simulink model "HLSDem_SelectParameter"  (R2016b)
settings: configuration reference "CodeGenConfigSet" (kept outside this file)
values from neighbouring files (symbols this model uses):
  HLSDem_facFdbkLoGrip_C = Calibration.Parameter    [init_HLSDem_SelectParameter.m]    (also in init_HLSDem_SelectParameter_SIL.m = Simulink.Parameter)
  HLSDem_facFdbkLoNoGrip_C = Calibration.Parameter    [init_HLSDem_SelectParameter.m]    (also in init_HLSDem_SelectParameter_SIL.m = Simulink.Parameter)
  HLSDem_facFdbkTrqLosHiGrip_CUR = Calibration.Parameter    [init_HLSDem_SelectParameter.m]    (also in init_HLSDem_SelectParameter_SIL.m = Simulink.Parameter)
  HLSDem_facFdbkTrqLosHiGrip_CURX = Calibration.Parameter    [init_HLSDem_SelectParameter.m]    (also in init_HLSDem_SelectParameter_SIL.m = Simulink.Parameter)
  HLSDem_facFdbkTrqLosHiNoGrip_C = Calibration.Parameter    [init_HLSDem_SelectParameter.m]    (also in init_HLSDem_SelectParameter_SIL.m = Simulink.Parameter)
  HLSDem_facFdbkTrqLosLoGrip_CUR = Calibration.Parameter    [init_HLSDem_SelectParameter.m]    (also in init_HLSDem_SelectParameter_SIL.m = Simulink.Parameter)
  HLSDem_facFdbkTrqLosLoGrip_CURX = Calibration.Parameter    [init_HLSDem_SelectParameter.m]    (also in init_HLSDem_SelectParameter_SIL.m = Simulink.Parameter)
  HLSDem_facFdbkTrqLosLoNoGrip_C = Calibration.Parameter    [init_HLSDem_SelectParameter.m]    (also in init_HLSDem_SelectParameter_SIL.m = Simulink.Parameter)
  HLSDem_facNAvrgPT1_C = Calibration.Parameter    [init_HLSDem_SelectParameter.m]    (also in init_HLSDem_SelectParameter_SIL.m = Simulink.Parameter)
  HLSDem_facTrqPT1CorFac_C = Calibration.Parameter    [init_HLSDem_SelectParameter.m]    (also in init_HLSDem_SelectParameter_SIL.m = Simulink.Parameter)
  HLSDem_GripIKiHi_CUR = Calibration.Parameter    [init_HLSDem_SelectParameter.m]    (also in init_HLSDem_SelectParameter_SIL.m = Simulink.Parameter)
  HLSDem_GripIKiHi_CURX = Calibration.Parameter    [init_HLSDem_SelectParameter.m]    (also in init_HLSDem_SelectParameter_SIL.m = Simulink.Parameter)
  HLSDem_GripIKiLo_CUR = Calibration.Parameter    [init_HLSDem_SelectParameter.m]    (also in init_HLSDem_SelectParameter_SIL.m = Simulink.Parameter)
  HLSDem_GripIKiLo_CURX = Calibration.Parameter    [init_HLSDem_SelectParameter.m]    (also in init_HLSDem_SelectParameter_SIL.m = Simulink.Parameter)
  HLSDem_GripIKiNegHi_CUR = Calibration.Parameter    [init_HLSDem_SelectParameter.m]    (also in init_HLSDem_SelectParameter_SIL.m = Simulink.Parameter)
  HLSDem_GripIKiNegHi_CURX = Calibration.Parameter    [init_HLSDem_SelectParameter.m]    (also in init_HLSDem_SelectParameter_SIL.m = Simulink.Parameter)
  HLSDem_GripIKiNegLo_CUR = Calibration.Parameter    [init_HLSDem_SelectParameter.m]    (also in init_HLSDem_SelectParameter_SIL.m = Simulink.Parameter)
  HLSDem_GripIKiNegLo_CURX = Calibration.Parameter    [init_HLSDem_SelectParameter.m]    (also in init_HLSDem_SelectParameter_SIL.m = Simulink.Parameter)
  HLSDem_GripIKiPosHi_CUR = Calibration.Parameter    [init_HLSDem_SelectParameter.m]    (also in init_HLSDem_SelectParameter_SIL.m = Simulink.Parameter)
  HLSDem_GripIKiPosHi_CURX = Calibration.Parameter    [init_HLSDem_SelectParameter.m]    (also in init_HLSDem_SelectParameter_SIL.m = Simulink.Parameter)
  HLSDem_GripIKiPosLo_CUR = Calibration.Parameter    [init_HLSDem_SelectParameter.m]    (also in init_HLSDem_SelectParameter_SIL.m = Simulink.Parameter)
  HLSDem_GripIKiPosLo_CURX = Calibration.Parameter    [init_HLSDem_SelectParameter.m]    (also in init_HLSDem_SelectParameter_SIL.m = Simulink.Parameter)
  HLSDem_GripIWinNegHi_C = Calibration.Parameter    [init_HLSDem_SelectParameter.m]    (also in init_HLSDem_SelectParameter_SIL.m = Simulink.Parameter)
  HLSDem_GripIWinNegLo_C = Calibration.Parameter    [init_HLSDem_SelectParameter.m]    (also in init_HLSDem_SelectParameter_SIL.m = Simulink.Parameter)
  HLSDem_GripIWinPosHi_C = Calibration.Parameter    [init_HLSDem_SelectParameter.m]    (also in init_HLSDem_SelectParameter_SIL.m = Simulink.Parameter)
  HLSDem_GripIWinPosLo_C = Calibration.Parameter    [init_HLSDem_SelectParameter.m]    (also in init_HLSDem_SelectParameter_SIL.m = Simulink.Parameter)
  HLSDem_GripPKpHi_CUR = Calibration.Parameter    [init_HLSDem_SelectParameter.m]    (also in init_HLSDem_SelectParameter_SIL.m = Simulink.Parameter)
  HLSDem_GripPKpHi_CURX = Calibration.Parameter    [init_HLSDem_SelectParameter.m]    (also in init_HLSDem_SelectParameter_SIL.m = Simulink.Parameter)
  HLSDem_GripPKpLo_CUR = Calibration.Parameter    [init_HLSDem_SelectParameter.m]    (also in init_HLSDem_SelectParameter_SIL.m = Simulink.Parameter)
  HLSDem_GripPKpLo_CURX = Calibration.Parameter    [init_HLSDem_SelectParameter.m]    (also in init_HLSDem_SelectParameter_SIL.m = Simulink.Parameter)
  HLSDem_GripPKpNegHi_CUR = Calibration.Parameter    [init_HLSDem_SelectParameter.m]    (also in init_HLSDem_SelectParameter_SIL.m = Simulink.Parameter)
  HLSDem_GripPKpNegHi_CURX = Calibration.Parameter    [init_HLSDem_SelectParameter.m]    (also in init_HLSDem_SelectParameter_SIL.m = Simulink.Parameter)
  HLSDem_GripPKpNegLo_CUR = Calibration.Parameter    [init_HLSDem_SelectParameter.m]    (also in init_HLSDem_SelectParameter_SIL.m = Simulink.Parameter)
  HLSDem_GripPKpNegLo_CURX = Calibration.Parameter    [init_HLSDem_SelectParameter.m]    (also in init_HLSDem_SelectParameter_SIL.m = Simulink.Parameter)
  HLSDem_GripPKpPosHi_CUR = Calibration.Parameter    [init_HLSDem_SelectParameter.m]    (also in init_HLSDem_SelectParameter_SIL.m = Simulink.Parameter)
  HLSDem_GripPKpPosHi_CURX = Calibration.Parameter    [init_HLSDem_SelectParameter.m]    (also in init_HLSDem_SelectParameter_SIL.m = Simulink.Parameter)
  HLSDem_GripPKpPosLo_CUR = Calibration.Parameter    [init_HLSDem_SelectParameter.m]    (also in init_HLSDem_SelectParameter_SIL.m = Simulink.Parameter)
  HLSDem_GripPKpPosLo_CURX = Calibration.Parameter    [init_HLSDem_SelectParameter.m]    (also in init_HLSDem_SelectParameter_SIL.m = Simulink.Parameter)
  HLSDem_GripPWinNegHi_C = Calibration.Parameter    [init_HLSDem_SelectParameter.m]    (also in init_HLSDem_SelectParameter_SIL.m = Simulink.Parameter)
  HLSDem_GripPWinNegLo_C = Calibration.Parameter    [init_HLSDem_SelectParameter.m]    (also in init_HLSDem_SelectParameter_SIL.m = Simulink.Parameter)
  HLSDem_GripPWinPosHi_C = Calibration.Parameter    [init_HLSDem_SelectParameter.m]    (also in init_HLSDem_SelectParameter_SIL.m = Simulink.Parameter)
  HLSDem_GripPWinPosLo_C = Calibration.Parameter    [init_HLSDem_SelectParameter.m]    (also in init_HLSDem_SelectParameter_SIL.m = Simulink.Parameter)
  HLSDem_InrtVehGrip_CUR = Calibration.Parameter    [init_HLSDem_SelectParameter.m]    (also in init_HLSDem_SelectParameter_SIL.m = Simulink.Parameter)
  HLSDem_InrtVehGrip_CURX = Calibration.Parameter    [init_HLSDem_SelectParameter.m]    (also in init_HLSDem_SelectParameter_SIL.m = Simulink.Parameter)
  HLSDem_InrtVehNoGrip_C = Calibration.Parameter    [init_HLSDem_SelectParameter.m]    (also in init_HLSDem_SelectParameter_SIL.m = Simulink.Parameter)
  HLSDem_KiCorFac_MAP = Calibration.Parameter    [init_HLSDem_SelectParameter.m]    (also in init_HLSDem_SelectParameter_SIL.m = Simulink.Parameter)
  HLSDem_KiCorFac_MAPX = Calibration.Parameter    [init_HLSDem_SelectParameter.m]    (also in init_HLSDem_SelectParameter_SIL.m = Simulink.Parameter)
  HLSDem_KiCorFac_MAPY = Calibration.Parameter    [init_HLSDem_SelectParameter.m]    (also in init_HLSDem_SelectParameter_SIL.m = Simulink.Parameter)
  HLSDem_KiCorTrqFac_MAP = Calibration.Parameter    [init_HLSDem_SelectParameter.m]    (also in init_HLSDem_SelectParameter_SIL.m = Simulink.Parameter)
  HLSDem_KiCorTrqFac_MAPX = Calibration.Parameter    [init_HLSDem_SelectParameter.m]    (also in init_HLSDem_SelectParameter_SIL.m = Simulink.Parameter)
  HLSDem_KiCorTrqFac_MAPY = Calibration.Parameter    [init_HLSDem_SelectParameter.m]    (also in init_HLSDem_SelectParameter_SIL.m = Simulink.Parameter)
  HLSDem_KpCorFac_MAP = Calibration.Parameter    [init_HLSDem_SelectParameter.m]    (also in init_HLSDem_SelectParameter_SIL.m = Simulink.Parameter)
  HLSDem_KpCorFac_MAPX = Calibration.Parameter    [init_HLSDem_SelectParameter.m]    (also in init_HLSDem_SelectParameter_SIL.m = Simulink.Parameter)
  HLSDem_KpCorFac_MAPY = Calibration.Parameter    [init_HLSDem_SelectParameter.m]    (also in init_HLSDem_SelectParameter_SIL.m = Simulink.Parameter)
  HLSDem_KpCorTrqFac_MAP = Calibration.Parameter    [init_HLSDem_SelectParameter.m]    (also in init_HLSDem_SelectParameter_SIL.m = Simulink.Parameter)
  HLSDem_KpCorTrqFac_MAPX = Calibration.Parameter    [init_HLSDem_SelectParameter.m]    (also in init_HLSDem_SelectParameter_SIL.m = Simulink.Parameter)
  HLSDem_KpCorTrqFac_MAPY = Calibration.Parameter    [init_HLSDem_SelectParameter.m]    (also in init_HLSDem_SelectParameter_SIL.m = Simulink.Parameter)
  HLSDem_NoGripdnAccLim_C = Calibration.Parameter    [init_HLSDem_SelectParameter.m]    (also in init_HLSDem_SelectParameter_SIL.m = Simulink.Parameter)
  HLSDem_NoGripdnDeclLim_C = Calibration.Parameter    [init_HLSDem_SelectParameter.m]    (also in init_HLSDem_SelectParameter_SIL.m = Simulink.Parameter)
  HLSDem_NoGripdnDeclLimBrk_C = Calibration.Parameter    [init_HLSDem_SelectParameter.m]    (also in init_HLSDem_SelectParameter_SIL.m = Simulink.Parameter)
  HLSDem_NoGripIKiHi_C = Calibration.Parameter    [init_HLSDem_SelectParameter.m]    (also in init_HLSDem_SelectParameter_SIL.m = Simulink.Parameter)
  HLSDem_NoGripIKiLo_C = Calibration.Parameter    [init_HLSDem_SelectParameter.m]    (also in init_HLSDem_SelectParameter_SIL.m = Simulink.Parameter)
  HLSDem_NoGripIKiNegHi_C = Calibration.Parameter    [init_HLSDem_SelectParameter.m]    (also in init_HLSDem_SelectParameter_SIL.m = Simulink.Parameter)
  HLSDem_NoGripIKiNegLo_C = Calibration.Parameter    [init_HLSDem_SelectParameter.m]    (also in init_HLSDem_SelectParameter_SIL.m = Simulink.Parameter)
  HLSDem_NoGripIKiPosHi_C = Calibration.Parameter    [init_HLSDem_SelectParameter.m]    (also in init_HLSDem_SelectParameter_SIL.m = Simulink.Parameter)
  HLSDem_NoGripIKiPosLo_C = Calibration.Parameter    [init_HLSDem_SelectParameter.m]    (also in init_HLSDem_SelectParameter_SIL.m = Simulink.Parameter)
  HLSDem_NoGripIWinNegHi_C = Calibration.Parameter    [init_HLSDem_SelectParameter.m]    (also in init_HLSDem_SelectParameter_SIL.m = Simulink.Parameter)
  HLSDem_NoGripIWinNegLo_C = Calibration.Parameter    [init_HLSDem_SelectParameter.m]    (also in init_HLSDem_SelectParameter_SIL.m = Simulink.Parameter)
  HLSDem_NoGripIWinPosHi_C = Calibration.Parameter    [init_HLSDem_SelectParameter.m]    (also in init_HLSDem_SelectParameter_SIL.m = Simulink.Parameter)
  HLSDem_NoGripIWinPosLo_C = Calibration.Parameter    [init_HLSDem_SelectParameter.m]    (also in init_HLSDem_SelectParameter_SIL.m = Simulink.Parameter)
  HLSDem_NoGripPKpHi_C = Calibration.Parameter    [init_HLSDem_SelectParameter.m]    (also in init_HLSDem_SelectParameter_SIL.m = Simulink.Parameter)
  HLSDem_NoGripPKpLo_C = Calibration.Parameter    [init_HLSDem_SelectParameter.m]    (also in init_HLSDem_SelectParameter_SIL.m = Simulink.Parameter)
  HLSDem_NoGripPKpNegHi_C = Calibration.Parameter    [init_HLSDem_SelectParameter.m]    (also in init_HLSDem_SelectParameter_SIL.m = Simulink.Parameter)
  HLSDem_NoGripPKpNegLo_C = Calibration.Parameter    [init_HLSDem_SelectParameter.m]    (also in init_HLSDem_SelectParameter_SIL.m = Simulink.Parameter)
  HLSDem_NoGripPKpPosHi_C = Calibration.Parameter    [init_HLSDem_SelectParameter.m]    (also in init_HLSDem_SelectParameter_SIL.m = Simulink.Parameter)
  HLSDem_NoGripPKpPosLo_C = Calibration.Parameter    [init_HLSDem_SelectParameter.m]    (also in init_HLSDem_SelectParameter_SIL.m = Simulink.Parameter)
  HLSDem_NoGripPWinNegHi_C = Calibration.Parameter    [init_HLSDem_SelectParameter.m]    (also in init_HLSDem_SelectParameter_SIL.m = Simulink.Parameter)
  HLSDem_NoGripPWinNegLo_C = Calibration.Parameter    [init_HLSDem_SelectParameter.m]    (also in init_HLSDem_SelectParameter_SIL.m = Simulink.Parameter)
  HLSDem_NoGripPWinPosHi_C = Calibration.Parameter    [init_HLSDem_SelectParameter.m]    (also in init_HLSDem_SelectParameter_SIL.m = Simulink.Parameter)
  HLSDem_NoGripPWinPosLo_C = Calibration.Parameter    [init_HLSDem_SelectParameter.m]    (also in init_HLSDem_SelectParameter_SIL.m = Simulink.Parameter)
  HLSDem_rNoGripThres_C = Calibration.Parameter    [init_HLSDem_SelectParameter.m]    (also in init_HLSDem_SelectParameter_SIL.m = Simulink.Parameter)
  HLSDem_stBrkTrq_C = Calibration.Parameter    [init_HLSDem_SelectParameter.m]    (also in init_HLSDem_SelectParameter_SIL.m = Simulink.Parameter)
  HLSDem_swtTempSelParAdap_C = Calibration.Parameter    [init_HLSDem_SelectParameter.m]    (also in init_HLSDem_SelectParameter_SIL.m = Simulink.Parameter)
  HLSDem_swtTrqSelCorFac_C = Calibration.Parameter    [init_HLSDem_SelectParameter.m]    (also in init_HLSDem_SelectParameter_SIL.m = Simulink.Parameter)
  HLSDem_tiFltTrqLosGrip_CUR = Calibration.Parameter    [init_HLSDem_SelectParameter.m]    (also in init_HLSDem_SelectParameter_SIL.m = Simulink.Parameter)
  HLSDem_tiFltTrqLosGrip_CURX = Calibration.Parameter    [init_HLSDem_SelectParameter.m]    (also in init_HLSDem_SelectParameter_SIL.m = Simulink.Parameter)
  HLSDem_tiFltTrqLosNoGrip_C = Calibration.Parameter    [init_HLSDem_SelectParameter.m]    (also in init_HLSDem_SelectParameter_SIL.m = Simulink.Parameter)
libraries: CXLib x2
(part 2 of 2)

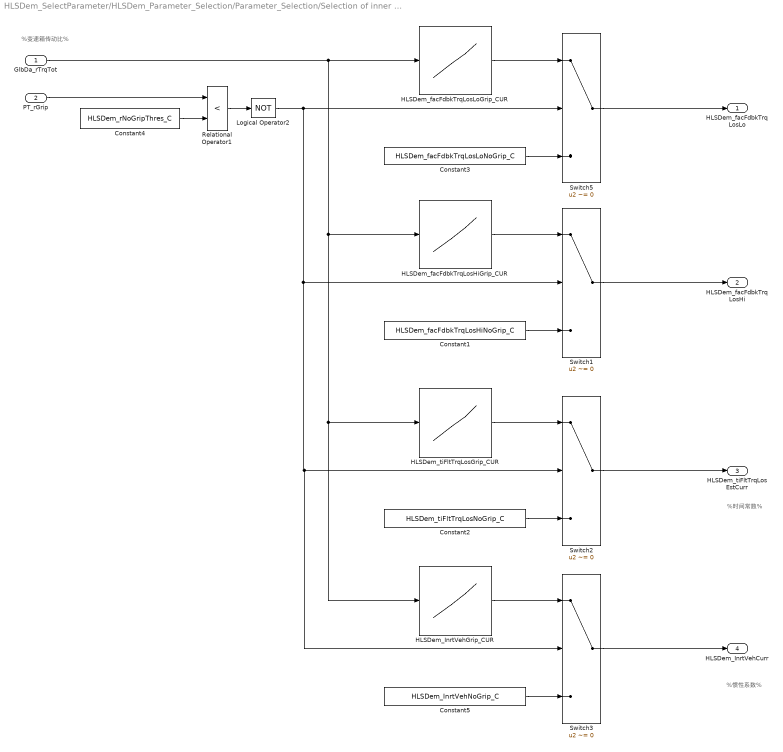
== system HLSDem_SelectParameter/HLSDem_Parameter_Selection/Parameter_Selection/Selection of inner feedback factor ==
  note: %时间常数%
  note: %变速箱传动比%
  note: %惯性系数%
  GlbDa_rTrqTot : Inport
  PT_rGrip : Inport  Port=2
  Constant1 : Constant  Value=HLSDem_facFdbkTrqLosHiNoGrip_C
  Constant2 : Constant  Value=HLSDem_tiFltTrqLosNoGrip_C
  Constant3 : Constant  Value=HLSDem_facFdbkTrqLosLoNoGrip_C
  Constant4 : Constant  Value=HLSDem_rNoGripThres_C
  Constant5 : Constant  Value=HLSDem_InrtVehNoGrip_C
  HLSDem_InrtVehGrip_CUR : Lookup_n-D  NumberOfTableDimensions=1  BreakpointsForDimension1=HLSDem_InrtVehGrip_CURX  BreakpointsForDimension2=HLSDem_KpCorFac_MAPX  Table=HLSDem_InrtVehGrip_CUR  ExtrapMethod=Clip  InternalRulePriority=Speed  OutDataTypeStr=Inherit: Inherit via back propagation  RndMeth=Simplest  SaturateOnIntegerOverflow=on
  HLSDem_facFdbkTrqLosHiGrip_CUR : Lookup_n-D  NumberOfTableDimensions=1  BreakpointsForDimension1=HLSDem_facFdbkTrqLosHiGrip_CURX  BreakpointsForDimension2=HLSDem_KpCorFac_MAPX  Table=HLSDem_facFdbkTrqLosHiGrip_CUR  ExtrapMethod=Clip  InternalRulePriority=Speed  OutDataTypeStr=Inherit: Inherit via back propagation  RndMeth=Simplest  SaturateOnIntegerOverflow=on
  HLSDem_facFdbkTrqLosLoGrip_CUR : Lookup_n-D  NumberOfTableDimensions=1  BreakpointsForDimension1=HLSDem_facFdbkTrqLosLoGrip_CURX  BreakpointsForDimension2=HLSDem_KpCorFac_MAPX  Table=HLSDem_facFdbkTrqLosLoGrip_CUR  ExtrapMethod=Clip  InternalRulePriority=Speed  OutDataTypeStr=Inherit: Inherit via back propagation  RndMeth=Simplest  SaturateOnIntegerOverflow=on
  HLSDem_tiFltTrqLosGrip_CUR : Lookup_n-D  NumberOfTableDimensions=1  BreakpointsForDimension1=HLSDem_tiFltTrqLosGrip_CURX  BreakpointsForDimension2=HLSDem_KpCorFac_MAPX  Table=HLSDem_tiFltTrqLosGrip_CUR  ExtrapMethod=Clip  InternalRulePriority=Speed  OutDataTypeStr=Inherit: Inherit via back propagation  RndMeth=Simplest  SaturateOnIntegerOverflow=on
  Logical Operator2 : Logic  Operator=NOT  AllPortsSameDT=off  OutDataTypeStr=boolean
  Relational Operator1 : RelationalOperator  Operator=<  OutDataTypeStr=boolean  RndMeth=Nearest  InputSameDT=on
  Switch{1..3,5} (4 alike) : Switch  Criteria=u2 ~= 0  InputSameDT=on
  HLSDem_facFdbkTrqLosLo : Outport
  HLSDem_facFdbkTrqLosHi : Outport  Port=2
  HLSDem_tiFltTrqLosEstCurr : Outport  Port=3
  HLSDem_InrtVehCurr : Outport  Port=4
  wires:
  Relational Operator1/1 -> Logical Operator2/1
  Switch2/1 -> HLSDem_tiFltTrqLosEstCurr/1
  GlbDa_rTrqTot/1 -> HLSDem_tiFltTrqLosGrip_CUR/1, HLSDem_InrtVehGrip_CUR/1, HLSDem_facFdbkTrqLosHiGrip_CUR/1, HLSDem_facFdbkTrqLosLoGrip_CUR/1
  Switch1/1 -> HLSDem_facFdbkTrqLosHi/1
  HLSDem_facFdbkTrqLosLoGrip_CUR/1 -> Switch5/1
  PT_rGrip/1 -> Relational Operator1/1
  HLSDem_facFdbkTrqLosHiGrip_CUR/1 -> Switch1/1
  Logical Operator2/1 -> Switch1/2, Switch3/2, Switch2/2, Switch5/2
  Constant3/1 -> Switch5/3
  Constant2/1 -> Switch2/3
  Constant1/1 -> Switch1/3
  Constant5/1 -> Switch3/3
  Switch5/1 -> HLSDem_facFdbkTrqLosLo/1
  HLSDem_tiFltTrqLosGrip_CUR/1 -> Switch2/1
  Constant4/1 -> Relational Operator1/2
  Switch3/1 -> HLSDem_InrtVehCurr/1
  HLSDem_InrtVehGrip_CUR/1 -> Switch3/1

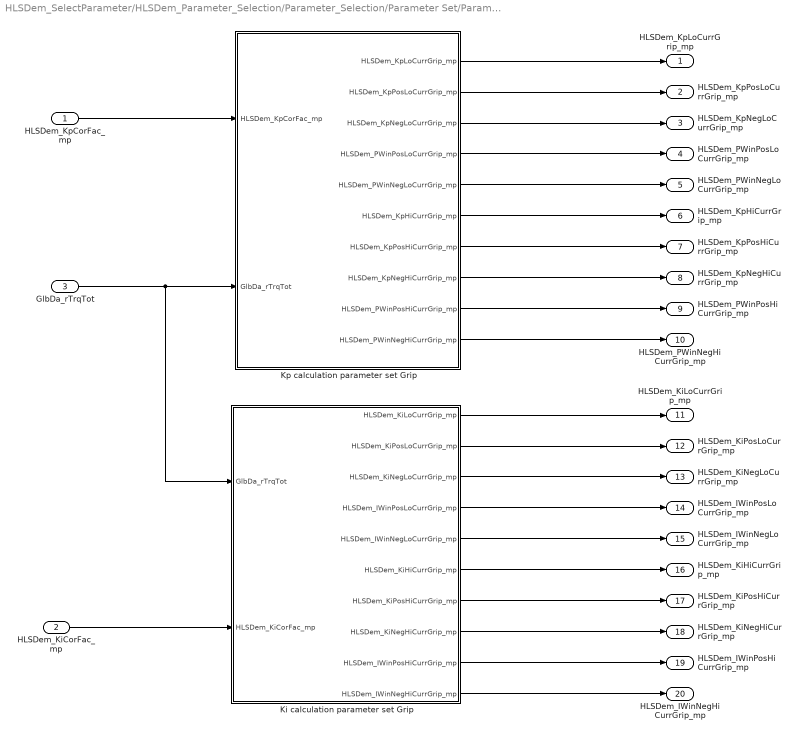
== system HLSDem_SelectParameter/HLSDem_Parameter_Selection/Parameter_Selection/Parameter Set/Parameter set Grip ==
  HLSDem_KpCorFac_mp : Inport
  HLSDem_KiCorFac_mp : Inport  Port=2
  GlbDa_rTrqTot : Inport  Port=3
  Ki calculation parameter set Grip : Subsystem
  Kp calculation parameter set Grip : Subsystem
  HLSDem_KpLoCurrGrip_mp : Outport
  HLSDem_KpPosLoCurrGrip_mp : Outport  Port=2
  HLSDem_KpNegLoCurrGrip_mp : Outport  Port=3
  HLSDem_PWinPosLoCurrGrip_mp : Outport  Port=4
  HLSDem_PWinNegLoCurrGrip_mp : Outport  Port=5
  HLSDem_KpHiCurrGrip_mp : Outport  Port=6
  HLSDem_KpPosHiCurrGrip_mp : Outport  Port=7
  HLSDem_KpNegHiCurrGrip_mp : Outport  Port=8
  HLSDem_PWinPosHiCurrGrip_mp : Outport  Port=9
  HLSDem_PWinNegHiCurrGrip_mp : Outport  Port=10
  HLSDem_KiLoCurrGrip_mp : Outport  Port=11
  HLSDem_KiPosLoCurrGrip_mp : Outport  Port=12
  HLSDem_KiNegLoCurrGrip_mp : Outport  Port=13
  HLSDem_IWinPosLoCurrGrip_mp : Outport  Port=14
  HLSDem_IWinNegLoCurrGrip_mp : Outport  Port=15
  HLSDem_KiHiCurrGrip_mp : Outport  Port=16
  HLSDem_KiPosHiCurrGrip_mp : Outport  Port=17
  HLSDem_KiNegHiCurrGrip_mp : Outport  Port=18
  HLSDem_IWinPosHiCurrGrip_mp : Outport  Port=19
  HLSDem_IWinNegHiCurrGrip_mp : Outport  Port=20
  wires:
  HLSDem_KiCorFac_mp/1 -> Ki calculation parameter set Grip/2(HLSDem_KiCorFac_mp)
  Ki calculation parameter set Grip/3(HLSDem_KiNegLoCurrGrip_mp) -> HLSDem_KiNegLoCurrGrip_mp/1
  Ki calculation parameter set Grip/5(HLSDem_IWinNegLoCurrGrip_mp) -> HLSDem_IWinNegLoCurrGrip_mp/1
  Ki calculation parameter set Grip/2(HLSDem_KiPosLoCurrGrip_mp) -> HLSDem_KiPosLoCurrGrip_mp/1
  Ki calculation parameter set Grip/4(HLSDem_IWinPosLoCurrGrip_mp) -> HLSDem_IWinPosLoCurrGrip_mp/1
  Kp calculation parameter set Grip/2(HLSDem_KpPosLoCurrGrip_mp) -> HLSDem_KpPosLoCurrGrip_mp/1
  Kp calculation parameter set Grip/7(HLSDem_KpPosHiCurrGrip_mp) -> HLSDem_KpPosHiCurrGrip_mp/1
  Kp calculation parameter set Grip/3(HLSDem_KpNegLoCurrGrip_mp) -> HLSDem_KpNegLoCurrGrip_mp/1
  Kp calculation parameter set Grip/6(HLSDem_KpHiCurrGrip_mp) -> HLSDem_KpHiCurrGrip_mp/1
  HLSDem_KpCorFac_mp/1 -> Kp calculation parameter set Grip/1(HLSDem_KpCorFac_mp)
  Kp calculation parameter set Grip/8(HLSDem_KpNegHiCurrGrip_mp) -> HLSDem_KpNegHiCurrGrip_mp/1
  Kp calculation parameter set Grip/5(HLSDem_PWinNegLoCurrGrip_mp) -> HLSDem_PWinNegLoCurrGrip_mp/1
  Kp calculation parameter set Grip/9(HLSDem_PWinPosHiCurrGrip_mp) -> HLSDem_PWinPosHiCurrGrip_mp/1
  Ki calculation parameter set Grip/9(HLSDem_IWinPosHiCurrGrip_mp) -> HLSDem_IWinPosHiCurrGrip_mp/1
  Ki calculation parameter set Grip/6(HLSDem_KiHiCurrGrip_mp) -> HLSDem_KiHiCurrGrip_mp/1
  Kp calculation parameter set Grip/4(HLSDem_PWinPosLoCurrGrip_mp) -> HLSDem_PWinPosLoCurrGrip_mp/1
  GlbDa_rTrqTot/1 -> Ki calculation parameter set Grip/1(GlbDa_rTrqTot), Kp calculation parameter set Grip/2(GlbDa_rTrqTot)
  Kp calculation parameter set Grip/1(HLSDem_KpLoCurrGrip_mp) -> HLSDem_KpLoCurrGrip_mp/1
  Ki calculation parameter set Grip/8(HLSDem_KiNegHiCurrGrip_mp) -> HLSDem_KiNegHiCurrGrip_mp/1
  Ki calculation parameter set Grip/10(HLSDem_IWinNegHiCurrGrip_mp) -> HLSDem_IWinNegHiCurrGrip_mp/1
  Ki calculation parameter set Grip/1(HLSDem_KiLoCurrGrip_mp) -> HLSDem_KiLoCurrGrip_mp/1
  Kp calculation parameter set Grip/10(HLSDem_PWinNegHiCurrGrip_mp) -> HLSDem_PWinNegHiCurrGrip_mp/1
  Ki calculation parameter set Grip/7(HLSDem_KiPosHiCurrGrip_mp) -> HLSDem_KiPosHiCurrGrip_mp/1

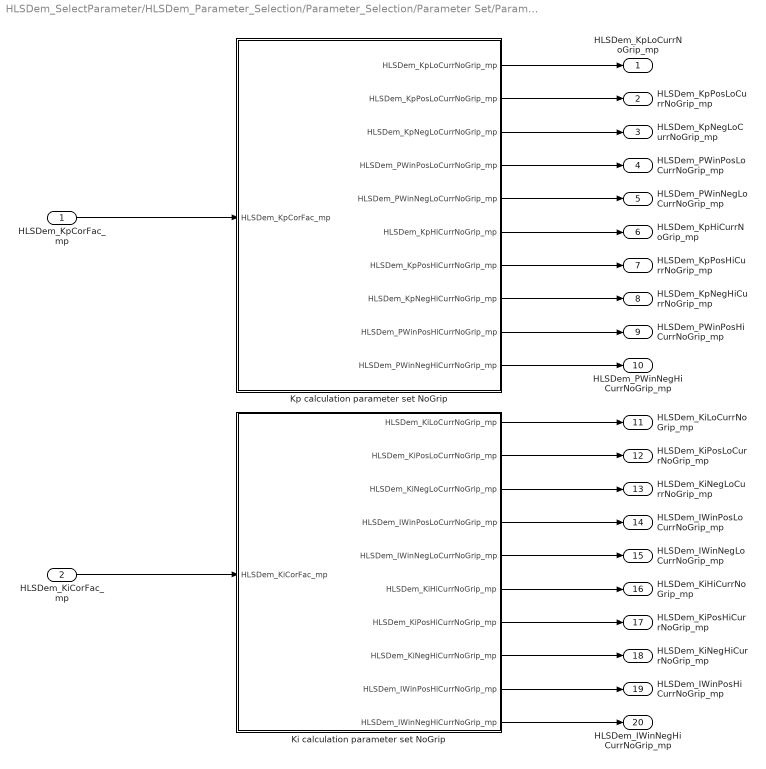
== system HLSDem_SelectParameter/HLSDem_Parameter_Selection/Parameter_Selection/Parameter Set/Parameter set NoGrip  ==
  HLSDem_KpCorFac_mp : Inport
  HLSDem_KiCorFac_mp : Inport  Port=2
  Ki calculation parameter set NoGrip : Subsystem
  Kp calculation parameter set NoGrip : Subsystem
  HLSDem_KpLoCurrNoGrip_mp : Outport
  HLSDem_KpPosLoCurrNoGrip_mp : Outport  Port=2
  HLSDem_KpNegLoCurrNoGrip_mp : Outport  Port=3
  HLSDem_PWinPosLoCurrNoGrip_mp : Outport  Port=4
  HLSDem_PWinNegLoCurrNoGrip_mp : Outport  Port=5
  HLSDem_KpHiCurrNoGrip_mp : Outport  Port=6
  HLSDem_KpPosHiCurrNoGrip_mp : Outport  Port=7
  HLSDem_KpNegHiCurrNoGrip_mp : Outport  Port=8
  HLSDem_PWinPosHiCurrNoGrip_mp : Outport  Port=9
  HLSDem_PWinNegHiCurrNoGrip_mp : Outport  Port=10
  HLSDem_KiLoCurrNoGrip_mp : Outport  Port=11
  HLSDem_KiPosLoCurrNoGrip_mp : Outport  Port=12
  HLSDem_KiNegLoCurrNoGrip_mp : Outport  Port=13
  HLSDem_IWinPosLoCurrNoGrip_mp : Outport  Port=14
  HLSDem_IWinNegLoCurrNoGrip_mp : Outport  Port=15
  HLSDem_KiHiCurrNoGrip_mp : Outport  Port=16
  HLSDem_KiPosHiCurrNoGrip_mp : Outport  Port=17
  HLSDem_KiNegHiCurrNoGrip_mp : Outport  Port=18
  HLSDem_IWinPosHiCurrNoGrip_mp : Outport  Port=19
  HLSDem_IWinNegHiCurrNoGrip_mp : Outport  Port=20
  wires:
  Kp calculation parameter set NoGrip/6(HLSDem_KpHiCurrNoGrip_mp) -> HLSDem_KpHiCurrNoGrip_mp/1
  Kp calculation parameter set NoGrip/7(HLSDem_KpPosHiCurrNoGrip_mp) -> HLSDem_KpPosHiCurrNoGrip_mp/1
  HLSDem_KpCorFac_mp/1 -> Kp calculation parameter set NoGrip/1(HLSDem_KpCorFac_mp)
  Kp calculation parameter set NoGrip/5(HLSDem_PWinNegLoCurrNoGrip_mp) -> HLSDem_PWinNegLoCurrNoGrip_mp/1
  Kp calculation parameter set NoGrip/9(HLSDem_PWinPosHiCurrNoGrip_mp) -> HLSDem_PWinPosHiCurrNoGrip_mp/1
  Kp calculation parameter set NoGrip/1(HLSDem_KpLoCurrNoGrip_mp) -> HLSDem_KpLoCurrNoGrip_mp/1
  Kp calculation parameter set NoGrip/3(HLSDem_KpNegLoCurrNoGrip_mp) -> HLSDem_KpNegLoCurrNoGrip_mp/1
  Kp calculation parameter set NoGrip/8(HLSDem_KpNegHiCurrNoGrip_mp) -> HLSDem_KpNegHiCurrNoGrip_mp/1
  HLSDem_KiCorFac_mp/1 -> Ki calculation parameter set NoGrip/1(HLSDem_KiCorFac_mp)
  Ki calculation parameter set NoGrip/10(HLSDem_IWinNegHiCurrNoGrip_mp) -> HLSDem_IWinNegHiCurrNoGrip_mp/1
  Ki calculation parameter set NoGrip/7(HLSDem_KiPosHiCurrNoGrip_mp) -> HLSDem_KiPosHiCurrNoGrip_mp/1
  Ki calculation parameter set NoGrip/9(HLSDem_IWinPosHiCurrNoGrip_mp) -> HLSDem_IWinPosHiCurrNoGrip_mp/1
  Kp calculation parameter set NoGrip/4(HLSDem_PWinPosLoCurrNoGrip_mp) -> HLSDem_PWinPosLoCurrNoGrip_mp/1
  Ki calculation parameter set NoGrip/8(HLSDem_KiNegHiCurrNoGrip_mp) -> HLSDem_KiNegHiCurrNoGrip_mp/1
  Ki calculation parameter set NoGrip/6(HLSDem_KiHiCurrNoGrip_mp) -> HLSDem_KiHiCurrNoGrip_mp/1
  Kp calculation parameter set NoGrip/2(HLSDem_KpPosLoCurrNoGrip_mp) -> HLSDem_KpPosLoCurrNoGrip_mp/1
  Ki calculation parameter set NoGrip/3(HLSDem_KiNegLoCurrNoGrip_mp) -> HLSDem_KiNegLoCurrNoGrip_mp/1
  Ki calculation parameter set NoGrip/4(HLSDem_IWinPosLoCurrNoGrip_mp) -> HLSDem_IWinPosLoCurrNoGrip_mp/1
  Ki calculation parameter set NoGrip/1(HLSDem_KiLoCurrNoGrip_mp) -> HLSDem_KiLoCurrNoGrip_mp/1
  Ki calculation parameter set NoGrip/2(HLSDem_KiPosLoCurrNoGrip_mp) -> HLSDem_KiPosLoCurrNoGrip_mp/1
  Kp calculation parameter set NoGrip/10(HLSDem_PWinNegHiCurrNoGrip_mp) -> HLSDem_PWinNegHiCurrNoGrip_mp/1
  Ki calculation parameter set NoGrip/5(HLSDem_IWinNegLoCurrNoGrip_mp) -> HLSDem_IWinNegLoCurrNoGrip_mp/1

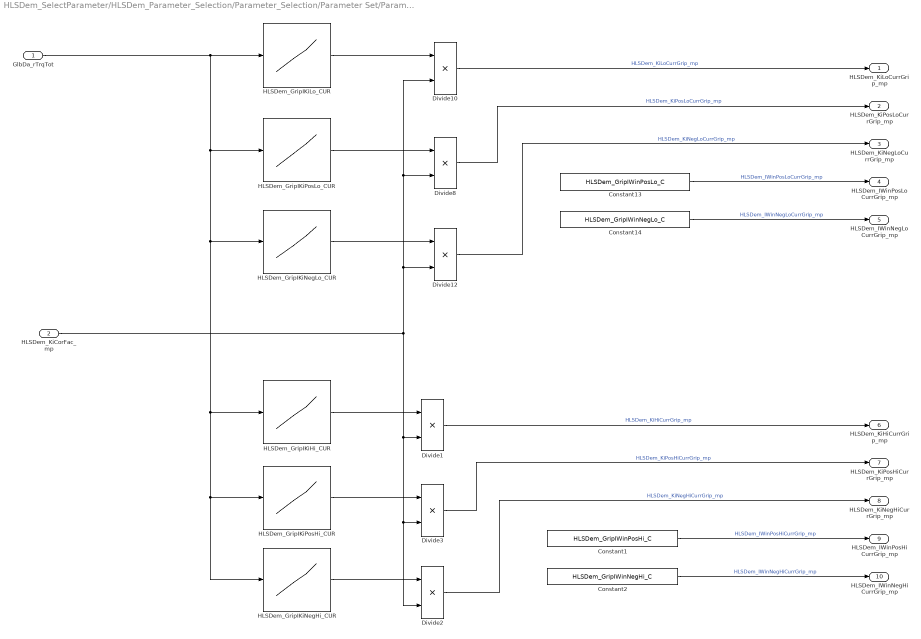
== system HLSDem_SelectParameter/HLSDem_Parameter_Selection/Parameter_Selection/Parameter Set/Parameter set Grip/Ki calculation parameter set Grip ==
  GlbDa_rTrqTot : Inport
  HLSDem_KiCorFac_mp : Inport  Port=2
  Constant1 : Constant  Value=HLSDem_GripIWinPosHi_C
  Constant13 : Constant  Value=HLSDem_GripIWinPosLo_C
  Constant14 : Constant  Value=HLSDem_GripIWinNegLo_C
  Constant2 : Constant  Value=HLSDem_GripIWinNegHi_C
  Divide{1..3,8,10,12} (6 alike) : Product  Inputs=**  OutDataTypeStr=HLSDem_Ki  SaturateOnIntegerOverflow=on
  HLSDem_GripIKiHi_CUR : Lookup_n-D  NumberOfTableDimensions=1  BreakpointsForDimension1=HLSDem_GripIKiHi_CURX  BreakpointsForDimension2=HLSDem_KpCorFac_MAPX  Table=HLSDem_GripIKiHi_CUR  ExtrapMethod=Clip  InternalRulePriority=Speed  OutDataTypeStr=Inherit: Inherit via back propagation  RndMeth=Simplest  SaturateOnIntegerOverflow=on
  HLSDem_GripIKiLo_CUR : Lookup_n-D  NumberOfTableDimensions=1  BreakpointsForDimension1=HLSDem_GripIKiLo_CURX  BreakpointsForDimension2=HLSDem_KpCorFac_MAPX  Table=HLSDem_GripIKiLo_CUR  ExtrapMethod=Clip  InternalRulePriority=Speed  OutDataTypeStr=Inherit: Inherit via back propagation  RndMeth=Simplest  SaturateOnIntegerOverflow=on
  HLSDem_GripIKiNegHi_CUR : Lookup_n-D  NumberOfTableDimensions=1  BreakpointsForDimension1=HLSDem_GripIKiNegHi_CURX  BreakpointsForDimension2=HLSDem_KpCorFac_MAPX  Table=HLSDem_GripIKiNegHi_CUR  ExtrapMethod=Clip  InternalRulePriority=Speed  OutDataTypeStr=Inherit: Inherit via back propagation  RndMeth=Simplest  SaturateOnIntegerOverflow=on
  HLSDem_GripIKiNegLo_CUR : Lookup_n-D  NumberOfTableDimensions=1  BreakpointsForDimension1=HLSDem_GripIKiNegLo_CURX  BreakpointsForDimension2=HLSDem_KpCorFac_MAPX  Table=HLSDem_GripIKiNegLo_CUR  ExtrapMethod=Clip  InternalRulePriority=Speed  OutDataTypeStr=Inherit: Inherit via back propagation  RndMeth=Simplest  SaturateOnIntegerOverflow=on
  HLSDem_GripIKiPosHi_CUR : Lookup_n-D  NumberOfTableDimensions=1  BreakpointsForDimension1=HLSDem_GripIKiPosHi_CURX  BreakpointsForDimension2=HLSDem_KpCorFac_MAPX  Table=HLSDem_GripIKiPosHi_CUR  ExtrapMethod=Clip  InternalRulePriority=Speed  OutDataTypeStr=Inherit: Inherit via back propagation  RndMeth=Simplest  SaturateOnIntegerOverflow=on
  HLSDem_GripIKiPosLo_CUR : Lookup_n-D  NumberOfTableDimensions=1  BreakpointsForDimension1=HLSDem_GripIKiPosLo_CURX  BreakpointsForDimension2=HLSDem_KpCorFac_MAPX  Table=HLSDem_GripIKiPosLo_CUR  ExtrapMethod=Clip  InternalRulePriority=Speed  OutDataTypeStr=Inherit: Inherit via back propagation  RndMeth=Simplest  SaturateOnIntegerOverflow=on
  HLSDem_KiLoCurrGrip_mp : Outport
  HLSDem_KiPosLoCurrGrip_mp : Outport  Port=2
  HLSDem_KiNegLoCurrGrip_mp : Outport  Port=3
  HLSDem_IWinPosLoCurrGrip_mp : Outport  Port=4
  HLSDem_IWinNegLoCurrGrip_mp : Outport  Port=5
  HLSDem_KiHiCurrGrip_mp : Outport  Port=6
  HLSDem_KiPosHiCurrGrip_mp : Outport  Port=7
  HLSDem_KiNegHiCurrGrip_mp : Outport  Port=8
  HLSDem_IWinPosHiCurrGrip_mp : Outport  Port=9
  HLSDem_IWinNegHiCurrGrip_mp : Outport  Port=10
  wires:
  HLSDem_GripIKiPosHi_CUR/1 -> Divide3/1
  HLSDem_GripIKiNegHi_CUR/1 -> Divide2/1
  HLSDem_GripIKiHi_CUR/1 -> Divide1/1
  Constant1/1 -> HLSDem_IWinPosHiCurrGrip_mp/1  "HLSDem_IWinPosHiCurrGrip_mp"
  Divide2/1 -> HLSDem_KiNegHiCurrGrip_mp/1  "HLSDem_KiNegHiCurrGrip_mp"
  Constant2/1 -> HLSDem_IWinNegHiCurrGrip_mp/1  "HLSDem_IWinNegHiCurrGrip_mp"
  GlbDa_rTrqTot/1 -> HLSDem_GripIKiPosLo_CUR/1, HLSDem_GripIKiNegHi_CUR/1, HLSDem_GripIKiPosHi_CUR/1, HLSDem_GripIKiHi_CUR/1, HLSDem_GripIKiNegLo_CUR/1, HLSDem_GripIKiLo_CUR/1
  Divide3/1 -> HLSDem_KiPosHiCurrGrip_mp/1  "HLSDem_KiPosHiCurrGrip_mp"
  Divide1/1 -> HLSDem_KiHiCurrGrip_mp/1  "HLSDem_KiHiCurrGrip_mp"
  Divide12/1 -> HLSDem_KiNegLoCurrGrip_mp/1  "HLSDem_KiNegLoCurrGrip_mp"
  Divide10/1 -> HLSDem_KiLoCurrGrip_mp/1  "HLSDem_KiLoCurrGrip_mp"
  HLSDem_GripIKiPosLo_CUR/1 -> Divide8/1
  Divide8/1 -> HLSDem_KiPosLoCurrGrip_mp/1  "HLSDem_KiPosLoCurrGrip_mp"
  Constant13/1 -> HLSDem_IWinPosLoCurrGrip_mp/1  "HLSDem_IWinPosLoCurrGrip_mp"
  Constant14/1 -> HLSDem_IWinNegLoCurrGrip_mp/1  "HLSDem_IWinNegLoCurrGrip_mp"
  HLSDem_GripIKiNegLo_CUR/1 -> Divide12/1
  HLSDem_KiCorFac_mp/1 -> Divide12/2, Divide8/2, Divide10/2, Divide2/2, Divide3/2, Divide1/2
  HLSDem_GripIKiLo_CUR/1 -> Divide10/1

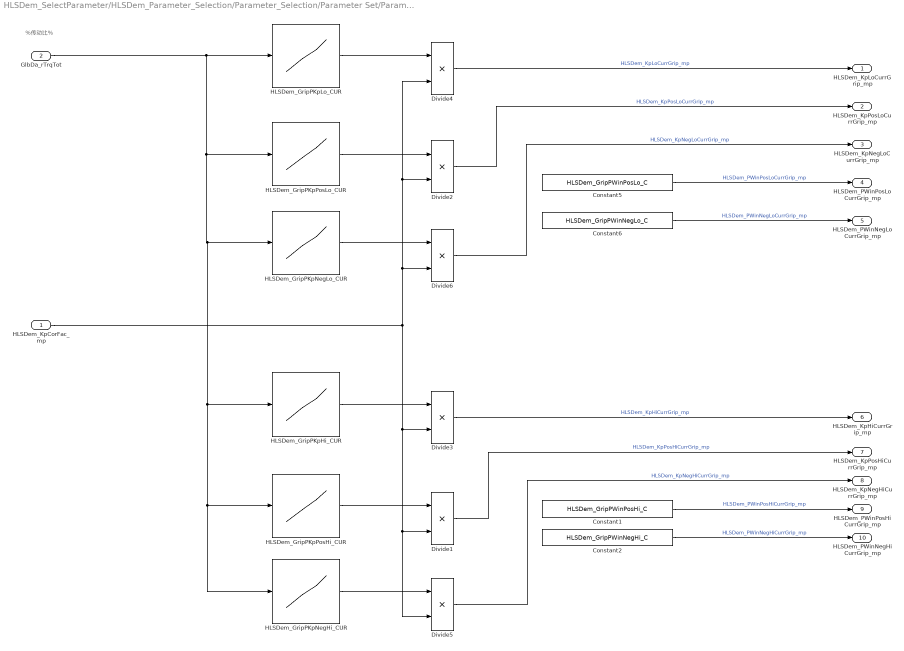
== system HLSDem_SelectParameter/HLSDem_Parameter_Selection/Parameter_Selection/Parameter Set/Parameter set Grip/Kp calculation parameter set Grip ==
  note: %传动比%
  HLSDem_KpCorFac_mp : Inport
  GlbDa_rTrqTot : Inport  Port=2
  Constant1 : Constant  Value=HLSDem_GripPWinPosHi_C
  Constant2 : Constant  Value=HLSDem_GripPWinNegHi_C
  Constant5 : Constant  Value=HLSDem_GripPWinPosLo_C
  Constant6 : Constant  Value=HLSDem_GripPWinNegLo_C
  Divide{1..6} (6 alike) : Product  Inputs=**  OutDataTypeStr=HLSDem_Kp  SaturateOnIntegerOverflow=on
  HLSDem_GripPKpHi_CUR : Lookup_n-D  NumberOfTableDimensions=1  BreakpointsForDimension1=HLSDem_GripPKpHi_CURX  BreakpointsForDimension2=HLSDem_KpCorFac_MAPX  Table=HLSDem_GripPKpHi_CUR  ExtrapMethod=Clip  InternalRulePriority=Speed  OutDataTypeStr=Inherit: Inherit via back propagation  RndMeth=Simplest  SaturateOnIntegerOverflow=on
  HLSDem_GripPKpLo_CUR : Lookup_n-D  NumberOfTableDimensions=1  BreakpointsForDimension1=HLSDem_GripPKpLo_CURX  BreakpointsForDimension2=HLSDem_KpCorFac_MAPX  Table=HLSDem_GripPKpLo_CUR  ExtrapMethod=Clip  InternalRulePriority=Speed  OutDataTypeStr=Inherit: Inherit via back propagation  RndMeth=Simplest  SaturateOnIntegerOverflow=on
  HLSDem_GripPKpNegHi_CUR : Lookup_n-D  NumberOfTableDimensions=1  BreakpointsForDimension1=HLSDem_GripPKpNegHi_CURX  BreakpointsForDimension2=HLSDem_KpCorFac_MAPX  Table=HLSDem_GripPKpNegHi_CUR  ExtrapMethod=Clip  InternalRulePriority=Speed  OutDataTypeStr=Inherit: Inherit via back propagation  RndMeth=Simplest  SaturateOnIntegerOverflow=on
  HLSDem_GripPKpNegLo_CUR : Lookup_n-D  NumberOfTableDimensions=1  BreakpointsForDimension1=HLSDem_GripPKpNegLo_CURX  BreakpointsForDimension2=HLSDem_KpCorFac_MAPX  Table=HLSDem_GripPKpNegLo_CUR  ExtrapMethod=Clip  InternalRulePriority=Speed  OutDataTypeStr=Inherit: Inherit via back propagation  RndMeth=Simplest  SaturateOnIntegerOverflow=on
  HLSDem_GripPKpPosHi_CUR : Lookup_n-D  NumberOfTableDimensions=1  BreakpointsForDimension1=HLSDem_GripPKpPosHi_CURX  BreakpointsForDimension2=HLSDem_KpCorFac_MAPX  Table=HLSDem_GripPKpPosHi_CUR  ExtrapMethod=Clip  InternalRulePriority=Speed  OutDataTypeStr=Inherit: Inherit via back propagation  RndMeth=Simplest  SaturateOnIntegerOverflow=on
  HLSDem_GripPKpPosLo_CUR : Lookup_n-D  NumberOfTableDimensions=1  BreakpointsForDimension1=HLSDem_GripPKpPosLo_CURX  BreakpointsForDimension2=HLSDem_KpCorFac_MAPX  Table=HLSDem_GripPKpPosLo_CUR  ExtrapMethod=Clip  InternalRulePriority=Speed  OutDataTypeStr=Inherit: Inherit via back propagation  RndMeth=Simplest  SaturateOnIntegerOverflow=on
  HLSDem_KpLoCurrGrip_mp : Outport
  HLSDem_KpPosLoCurrGrip_mp : Outport  Port=2
  HLSDem_KpNegLoCurrGrip_mp : Outport  Port=3
  HLSDem_PWinPosLoCurrGrip_mp : Outport  Port=4
  HLSDem_PWinNegLoCurrGrip_mp : Outport  Port=5
  HLSDem_KpHiCurrGrip_mp : Outport  Port=6
  HLSDem_KpPosHiCurrGrip_mp : Outport  Port=7
  HLSDem_KpNegHiCurrGrip_mp : Outport  Port=8
  HLSDem_PWinPosHiCurrGrip_mp : Outport  Port=9
  HLSDem_PWinNegHiCurrGrip_mp : Outport  Port=10
  wires:
  Constant2/1 -> HLSDem_PWinNegHiCurrGrip_mp/1  "HLSDem_PWinNegHiCurrGrip_mp"
  HLSDem_GripPKpPosHi_CUR/1 -> Divide1/1
  Divide2/1 -> HLSDem_KpPosLoCurrGrip_mp/1  "HLSDem_KpPosLoCurrGrip_mp"
  HLSDem_KpCorFac_mp/1 -> Divide4/2, Divide2/2, Divide6/2, Divide5/2, Divide1/2, Divide3/2
  HLSDem_GripPKpHi_CUR/1 -> Divide3/1
  GlbDa_rTrqTot/1 -> HLSDem_GripPKpHi_CUR/1, HLSDem_GripPKpPosHi_CUR/1, HLSDem_GripPKpNegHi_CUR/1, HLSDem_GripPKpNegLo_CUR/1, HLSDem_GripPKpPosLo_CUR/1, HLSDem_GripPKpLo_CUR/1
  HLSDem_GripPKpNegHi_CUR/1 -> Divide5/1
  Constant6/1 -> HLSDem_PWinNegLoCurrGrip_mp/1  "HLSDem_PWinNegLoCurrGrip_mp"
  Divide3/1 -> HLSDem_KpHiCurrGrip_mp/1  "HLSDem_KpHiCurrGrip_mp"
  Constant1/1 -> HLSDem_PWinPosHiCurrGrip_mp/1  "HLSDem_PWinPosHiCurrGrip_mp"
  Divide1/1 -> HLSDem_KpPosHiCurrGrip_mp/1  "HLSDem_KpPosHiCurrGrip_mp"
  Divide6/1 -> HLSDem_KpNegLoCurrGrip_mp/1  "HLSDem_KpNegLoCurrGrip_mp"
  HLSDem_GripPKpPosLo_CUR/1 -> Divide2/1
  HLSDem_GripPKpLo_CUR/1 -> Divide4/1
  Divide5/1 -> HLSDem_KpNegHiCurrGrip_mp/1  "HLSDem_KpNegHiCurrGrip_mp"
  HLSDem_GripPKpNegLo_CUR/1 -> Divide6/1
  Constant5/1 -> HLSDem_PWinPosLoCurrGrip_mp/1  "HLSDem_PWinPosLoCurrGrip_mp"
  Divide4/1 -> HLSDem_KpLoCurrGrip_mp/1  "HLSDem_KpLoCurrGrip_mp"

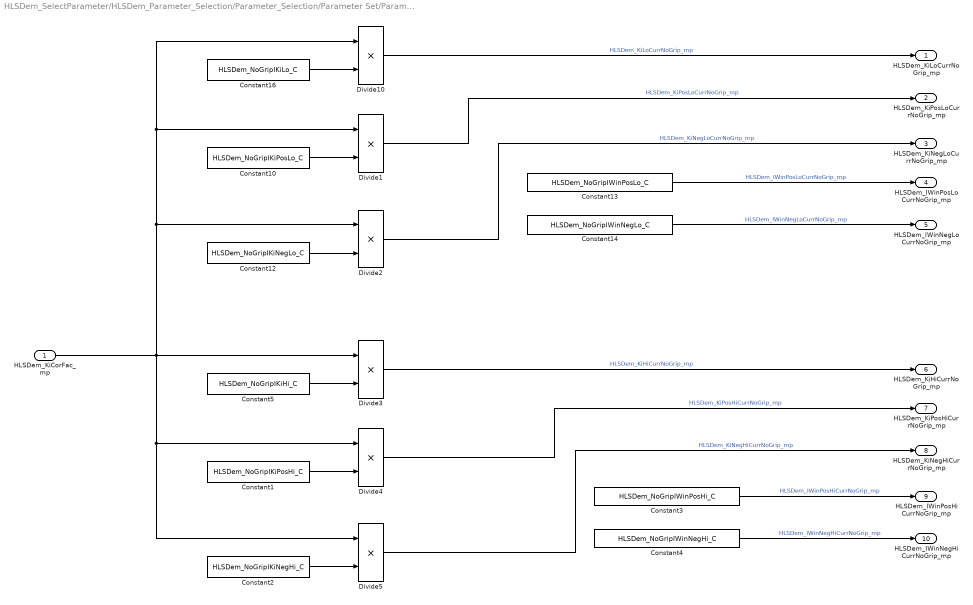
== system HLSDem_SelectParameter/HLSDem_Parameter_Selection/Parameter_Selection/Parameter Set/Parameter set NoGrip /Ki calculation parameter set NoGrip ==
  HLSDem_KiCorFac_mp : Inport
  Constant1 : Constant  Value=HLSDem_NoGripIKiPosHi_C
  Constant10 : Constant  Value=HLSDem_NoGripIKiPosLo_C
  Constant12 : Constant  Value=HLSDem_NoGripIKiNegLo_C
  Constant13 : Constant  Value=HLSDem_NoGripIWinPosLo_C
  Constant14 : Constant  Value=HLSDem_NoGripIWinNegLo_C
  Constant16 : Constant  Value=HLSDem_NoGripIKiLo_C
  Constant2 : Constant  Value=HLSDem_NoGripIKiNegHi_C
  Constant3 : Constant  Value=HLSDem_NoGripIWinPosHi_C
  Constant4 : Constant  Value=HLSDem_NoGripIWinNegHi_C
  Constant5 : Constant  Value=HLSDem_NoGripIKiHi_C
  Divide{1..5,10} (6 alike) : Product  Inputs=**  OutDataTypeStr=Inherit: Inherit via back propagation  RndMeth=Round  SaturateOnIntegerOverflow=on
  HLSDem_KiLoCurrNoGrip_mp : Outport
  HLSDem_KiPosLoCurrNoGrip_mp : Outport  Port=2
  HLSDem_KiNegLoCurrNoGrip_mp : Outport  Port=3
  HLSDem_IWinPosLoCurrNoGrip_mp : Outport  Port=4
  HLSDem_IWinNegLoCurrNoGrip_mp : Outport  Port=5
  HLSDem_KiHiCurrNoGrip_mp : Outport  Port=6
  HLSDem_KiPosHiCurrNoGrip_mp : Outport  Port=7
  HLSDem_KiNegHiCurrNoGrip_mp : Outport  Port=8
  HLSDem_IWinPosHiCurrNoGrip_mp : Outport  Port=9
  HLSDem_IWinNegHiCurrNoGrip_mp : Outport  Port=10
  wires:
  Constant16/1 -> Divide10/2
  Constant10/1 -> Divide1/2
  Divide10/1 -> HLSDem_KiLoCurrNoGrip_mp/1  "HLSDem_KiLoCurrNoGrip_mp"
  Constant4/1 -> HLSDem_IWinNegHiCurrNoGrip_mp/1  "HLSDem_IWinNegHiCurrNoGrip_mp"
  Divide2/1 -> HLSDem_KiNegLoCurrNoGrip_mp/1  "HLSDem_KiNegLoCurrNoGrip_mp"
  Constant12/1 -> Divide2/2
  Divide1/1 -> HLSDem_KiPosLoCurrNoGrip_mp/1  "HLSDem_KiPosLoCurrNoGrip_mp"
  Constant14/1 -> HLSDem_IWinNegLoCurrNoGrip_mp/1  "HLSDem_IWinNegLoCurrNoGrip_mp"
  HLSDem_KiCorFac_mp/1 -> Divide3/1, Divide2/1, Divide1/1, Divide10/1, Divide5/1, Divide4/1
  Constant5/1 -> Divide3/2
  Constant1/1 -> Divide4/2
  Constant2/1 -> Divide5/2
  Divide3/1 -> HLSDem_KiHiCurrNoGrip_mp/1  "HLSDem_KiHiCurrNoGrip_mp"
  Divide4/1 -> HLSDem_KiPosHiCurrNoGrip_mp/1  "HLSDem_KiPosHiCurrNoGrip_mp"
  Divide5/1 -> HLSDem_KiNegHiCurrNoGrip_mp/1  "HLSDem_KiNegHiCurrNoGrip_mp"
  Constant3/1 -> HLSDem_IWinPosHiCurrNoGrip_mp/1  "HLSDem_IWinPosHiCurrNoGrip_mp"
  Constant13/1 -> HLSDem_IWinPosLoCurrNoGrip_mp/1  "HLSDem_IWinPosLoCurrNoGrip_mp"

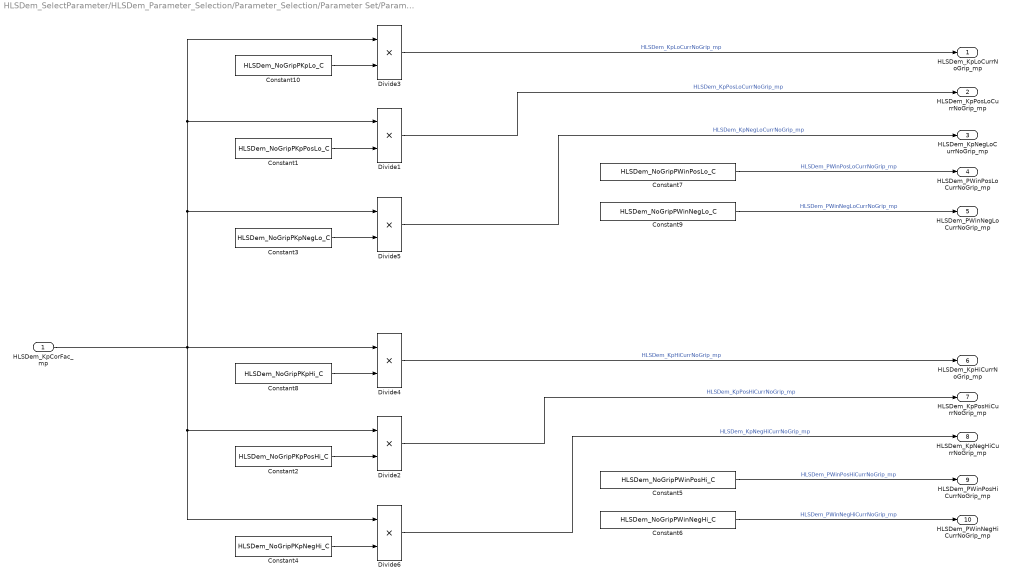
== system HLSDem_SelectParameter/HLSDem_Parameter_Selection/Parameter_Selection/Parameter Set/Parameter set NoGrip /Kp calculation parameter set NoGrip ==
  HLSDem_KpCorFac_mp : Inport
  Constant1 : Constant  Value=HLSDem_NoGripPKpPosLo_C
  Constant10 : Constant  Value=HLSDem_NoGripPKpLo_C
  Constant2 : Constant  Value=HLSDem_NoGripPKpPosHi_C
  Constant3 : Constant  Value=HLSDem_NoGripPKpNegLo_C
  Constant4 : Constant  Value=HLSDem_NoGripPKpNegHi_C
  Constant5 : Constant  Value=HLSDem_NoGripPWinPosHi_C
  Constant6 : Constant  Value=HLSDem_NoGripPWinNegHi_C
  Constant7 : Constant  Value=HLSDem_NoGripPWinPosLo_C
  Constant8 : Constant  Value=HLSDem_NoGripPKpHi_C
  Constant9 : Constant  Value=HLSDem_NoGripPWinNegLo_C
  Divide{1..6} (6 alike) : Product  Inputs=**  OutDataTypeStr=Inherit: Inherit via back propagation  RndMeth=Round  SaturateOnIntegerOverflow=on
  HLSDem_KpLoCurrNoGrip_mp : Outport
  HLSDem_KpPosLoCurrNoGrip_mp : Outport  Port=2
  HLSDem_KpNegLoCurrNoGrip_mp : Outport  Port=3
  HLSDem_PWinPosLoCurrNoGrip_mp : Outport  Port=4
  HLSDem_PWinNegLoCurrNoGrip_mp : Outport  Port=5
  HLSDem_KpHiCurrNoGrip_mp : Outport  Port=6
  HLSDem_KpPosHiCurrNoGrip_mp : Outport  Port=7
  HLSDem_KpNegHiCurrNoGrip_mp : Outport  Port=8
  HLSDem_PWinPosHiCurrNoGrip_mp : Outport  Port=9
  HLSDem_PWinNegHiCurrNoGrip_mp : Outport  Port=10
  wires:
  HLSDem_KpCorFac_mp/1 -> Divide6/1, Divide2/1, Divide3/1, Divide1/1, Divide5/1, Divide4/1
  Constant10/1 -> Divide3/2
  Constant1/1 -> Divide1/2
  Constant3/1 -> Divide5/2
  Divide3/1 -> HLSDem_KpLoCurrNoGrip_mp/1  "HLSDem_KpLoCurrNoGrip_mp"
  Divide1/1 -> HLSDem_KpPosLoCurrNoGrip_mp/1  "HLSDem_KpPosLoCurrNoGrip_mp"
  Divide5/1 -> HLSDem_KpNegLoCurrNoGrip_mp/1  "HLSDem_KpNegLoCurrNoGrip_mp"
  Constant7/1 -> HLSDem_PWinPosLoCurrNoGrip_mp/1  "HLSDem_PWinPosLoCurrNoGrip_mp"
  Constant5/1 -> HLSDem_PWinPosHiCurrNoGrip_mp/1  "HLSDem_PWinPosHiCurrNoGrip_mp"
  Constant9/1 -> HLSDem_PWinNegLoCurrNoGrip_mp/1  "HLSDem_PWinNegLoCurrNoGrip_mp"
  Divide6/1 -> HLSDem_KpNegHiCurrNoGrip_mp/1  "HLSDem_KpNegHiCurrNoGrip_mp"
  Constant6/1 -> HLSDem_PWinNegHiCurrNoGrip_mp/1  "HLSDem_PWinNegHiCurrNoGrip_mp"
  Divide4/1 -> HLSDem_KpHiCurrNoGrip_mp/1  "HLSDem_KpHiCurrNoGrip_mp"
  Constant8/1 -> Divide4/2
  Divide2/1 -> HLSDem_KpPosHiCurrNoGrip_mp/1  "HLSDem_KpPosHiCurrNoGrip_mp"
  Constant2/1 -> Divide2/2
  Constant4/1 -> Divide6/2
